simulink model "reference_filter_1_6"  (R2020b)
settings: Solver=VariableStepAuto  StartTime=0.0  StopTime=10.0  MaxStep=0.001  RelTol=1e-3
settings Model: Creator=Lenovo  LastModifiedBy=Lenovo
settings DataIOCC: SaveOutput=off  SaveTime=off

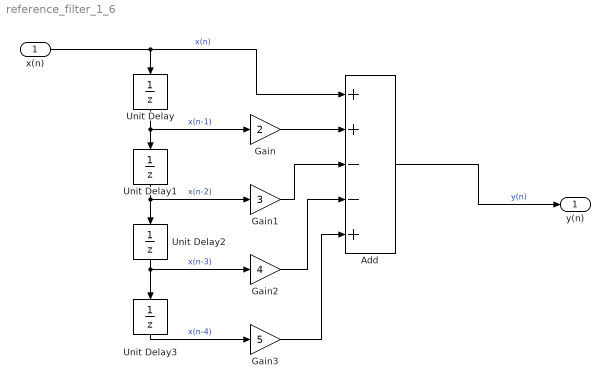
== system reference_filter_1_6 ==
  x(n) : Inport  OutDataTypeStr=double  PortDimensions=1  SampleTime=0
  Add : Sum  Inputs=++--+
  Gain : Gain  Gain=2
  Gain1 : Gain  Gain=3
  Gain2 : Gain  Gain=4
  Gain3 : Gain  Gain=5
  Unit Delay{,1..3} (4 alike) : UnitDelay  SampleTime=-1  HasFrameUpgradeWarning=on
  y(n) : Outport  OutDataTypeStr=double  PortDimensions=1  SampleTime=0
  wires:
  Unit Delay/1 -> Gain/1, Unit Delay1/1  "x(n-1)"
  Unit Delay1/1 -> Gain1/1, Unit Delay2/1  "x(n-2)"
  x(n)/1 -> Add/1, Unit Delay/1  "x(n)"
  Gain1/1 -> Add/3
  Unit Delay3/1 -> Gain3/1  "x(n-4)"
  Unit Delay2/1 -> Gain2/1, Unit Delay3/1  "x(n-3)"
  Gain2/1 -> Add/4
  Gain3/1 -> Add/5
  Gain/1 -> Add/2
  Add/1 -> y(n)/1  "y(n)"
